simulink model "RCAM_OP_LAT"  (R2022b)
settings: Solver=VariableStepAuto  StartTime=0.0  StopTime=TF  RelTol=1e-3
undefined symbols (not defined in the file): id_lat, X0
libraries: cstblocks x1
settings Model: Creator=bendr  LastModifiedBy=bendr

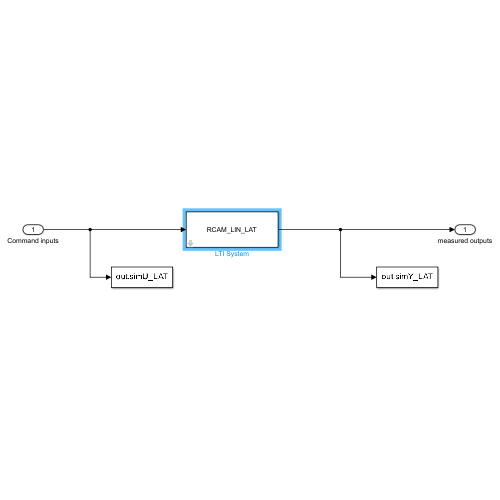
[thumbnail: Simulink's stored preview of the top-level diagram]
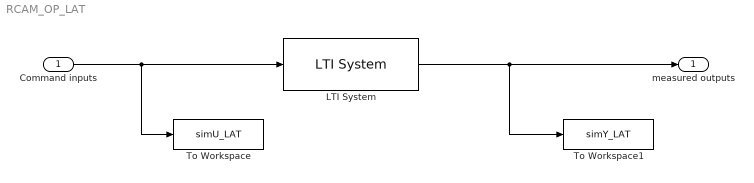
== system RCAM_OP_LAT ==
  Command inputs : Inport  PortDimensions=5
  LTI System : cstblocks/LTI System  sys=RCAM_LIN_LAT  IC=X0(id_lat)
  To Workspace : ToWorkspace  VariableName=simU_LAT  SaveFormat=Timeseries  SampleTime=-1
  To Workspace1 : ToWorkspace  VariableName=simY_LAT  SaveFormat=Timeseries  SampleTime=-1
  measured outputs : Outport
  wires:
  Command inputs/1 -> To Workspace/1, LTI System/1
  LTI System/1 -> To Workspace1/1, measured outputs/1
